simulink library "tqr"  (R2021b)
settings: Solver=VariableStepAuto  StartTime=0.0  StopTime=10.0  RelTol=1e-3
undefined symbols (not defined in the file or in its folder): ATQR_AltRDCActiveFEDUInc_X_pct, ATQR_AltRDCActiveFEDUInc_Y_enum, ATQR_AltRDCActiveFEDUTs_X_pct, ATQR_AltRDCActiveFEDUTs_Y_enum, ATQR_AltRDCActiveREDUInc_X_pct, ATQR_AltRDCActiveREDUInc_Y_enum, ATQR_AltRDCActiveREDUTs_X_pct, ATQR_AltRDCActiveREDUTs_Y_enum, ATQR_CreepFEDUTqIncSR_X_rpm, ATQR_CreepFEDUTqIncSR_Y_Nm, ATQR_CreepFEDUTs_X_rpm, ATQR_CreepFEDUTs_Y_Nm, ATQR_EcoTqFrIncGain_X_Nm, ATQR_EcoTqFrIncGain_Y_pct, ATQR_EcoTqRrIncGain_X_Nm, ATQR_EcoTqRrIncGain_Y_pct, ATQR_EL1FEDUTqDecSR_Y_Nm, ATQR_EL1FEDUTqIncSR_X_rpm, ATQR_EL1FEDUTqIncSR_Y_pct, ATQR_EL1FEDUTs_X_rpm, ATQR_EL1FEDUTs_Y_Nm, ATQR_EL1REDUTqDecSR_Y_Nm, ATQR_EL1REDUTs_Y_Nm, ATQR_FEDUEL1RegenTs_X_rpm, ATQR_FEDUTIPOutTs_X_rpm, ATQR_FrNegRateLimitIncN_X_rpm, ATQR_FrNegRateLimitIncN_Y_Nm, ATQR_FrPosRateLimitIncN_X_rpm, ATQR_FrPosRateLimitIncN_Y_Nm, ATQR_FShaftSpdTqLimCoe_X_rpm, ATQR_FTimerTqLimCoe_X_s, ATQR_FTqZeroTransUpBoundN_X_rpm, ATQR_NL1FEDUTqDecSR_Y_Nm, ATQR_NL1FEDUTqIncSR_X_rpm, ATQR_NL1FEDUTqIncSR_Y_pct, ATQR_NL1FEDUTs_X_rpm, ATQR_NL1FEDUTs_Y_Nm, ATQR_NL1REDUTqDecSR_Y_Nm, ATQR_NL1REDUTs_Y_Nm, ATQR_NormalTqFrIncGain_X_Nm, ATQR_NormalTqFrIncGain_Y_pct, ATQR_NormalTqRrIncGain_X_Nm, ATQR_NormalTqRrIncGain_Y_pct, ATQR_RrNegRateLimitIncN_X_rpm, ATQR_RrNegRateLimitIncN_Y_Nm, ATQR_RrPosRateLimitIncN_X_rpm, ATQR_RrPosRateLimitIncN_Y_Nm, ATQR_RShaftSpdTqLimCoe_X_rpm, ATQR_RTimerTqLimCoe_X_s, ATQR_SL1FEDUTqDecSR_Y_Nm, ATQR_SL1FEDUTqIncSR_X_rpm, ATQR_SL1FEDUTqIncSR_Y_pct, ATQR_SL1FEDUTs_X_rpm, ATQR_SL1FEDUTs_Y_Nm, ATQR_SL1REDUTqDecSR_Y_Nm, ATQR_SL1REDUTs_Y_Nm, ATQR_SportTqFrIncGain_X_Nm, ATQR_SportTqFrIncGain_Y_pct, ATQR_SportTqRrIncGain_X_Nm, ATQR_SportTqRrIncGain_Y_pct ... (+287)
libraries: hcu_lib x19, simulink x17, $bdroot x3
(part 3 of 10)

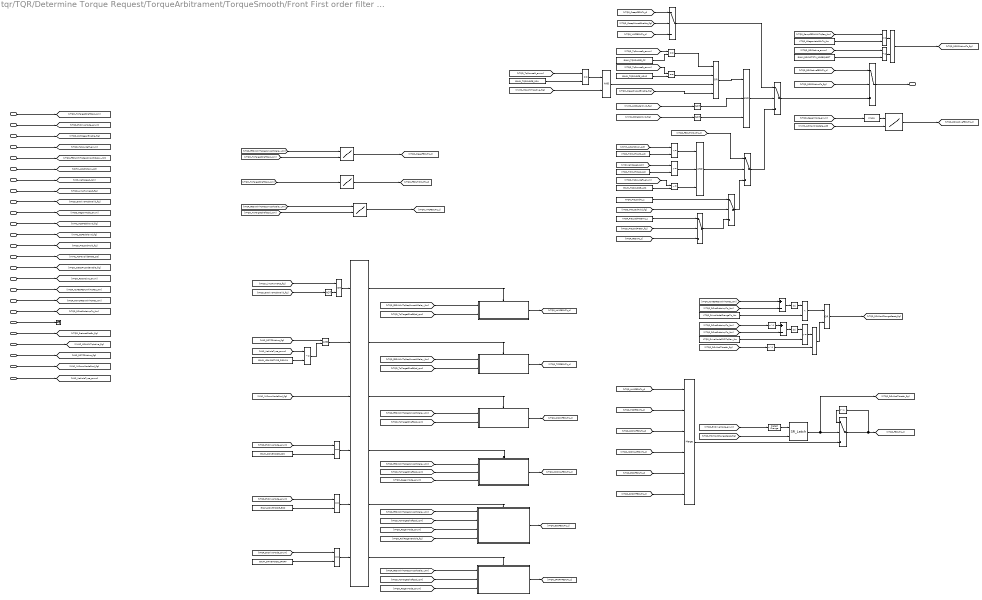
== system tqr/TQR/Determine Torque Request/TorqueArbitrament/TorqueSmooth/Front First order filter input tau map and determination ==
  VTQD_TqTargetShaftSpd_rpm : Inport
  VTQR_EVDriveMode_enum : Inport  Port=2
  VTQD_RollRegenEnable_flg : Inport  Port=3
  VTQD_TqSourceFr_enum : Inport  Port=4
  VTQR_FEDUWhlTqReqSmoothDelay_Nm : Inport  Port=5
  VDHP_ActAPSPosn_pct : Inport  Port=6
  VINP_VehSpeed_kph : Inport  Port=7
  VTQD_LimpHomeAct_flg : Inport  Port=8
  VTQD_EVDriveModeValid_flg : Inport  Port=9
  VTQD_RegenMode_enum : Inport  Port=10
  VVMC_ACCPedalOvrd_flg : Inport  Port=11
  VVMC_CCPedalOvrd_flg : Inport  Port=12
  VTQD_PreLoadHold_flg : Inport  Port=13
  VVMC_ActMaxSlideRate_pct : Inport  Port=14
  VTQD_CreepPrLoadEnable_flg : Inport  Port=15
  VTQD_RDCActive_enum : Inport  Port=16
  VTQR_NoABSFEDUWhlTqReq_Nm : Inport  Port=17
  VTQR_RampFEDUWhlTqReq_Nm : Inport  Port=18
  VTQR_FrFirstOrderInpTq_Nm : Inport  Port=19
  VTQD_PedAccTqEn_flg : Inport  Port=20
  VTQD_PreLoadPreEn_flg : Inport  Port=21
  VVMC_MSAWhlTqActive_flg : Inport  Port=22
  VINP_FrPTCSActive_flg : Inport  Port=23
  VINP_IVISnowModeCmd_flg : Inport  Port=24
  VINP_VehicleType_enum : Inport  Port=25
  AND : Logic  AllPortsSameDT=off  OutDataTypeStr=boolean
  AND1 : Logic  Inputs=3  AllPortsSameDT=off  OutDataTypeStr=boolean
  AND2 : Logic  Inputs=3  AllPortsSameDT=off  OutDataTypeStr=boolean
  AND3 : Logic  AllPortsSameDT=off  OutDataTypeStr=boolean
  AND4 : Logic  AllPortsSameDT=off  OutDataTypeStr=boolean
  Abs : Abs
  Abs4 : Abs
  Add : Sum  Inputs=+-
  Add1 : Sum  Inputs=+-
  Constant : Constant  Value=ENUM_VEHICLETYPE_D31L24
  Constant1 : Constant  Value=ENUM_TQSOURCE_APS
  Constant11 : Constant  Value=ENUM_DRIVEMODE_ECO
  Constant12 : Constant  Value=ENUM_DRIVEMODE_NRM
  Constant16 : Constant  Value=ENUM_DRIVEMODE_SPORT
  Constant2 : Constant  Value=KTQR_DriveModeCMDTqDev_Nm
  Constant3 : Constant  Value=ENUM_TQSOURCE_CC
  Constant32 : Constant  Value=KTQR_TIPOutTsAPS_pct
  Constant33 : Constant  Value=KTQR_TIPOutTsSpd_kph
  Constant34 : Constant  Value=ENUM_TQSOURCE_ADAS
  Constant4 : Constant  Value=KTQR_PreLoadTs_c
  Constant5 : Constant  Value=KTQR_ARegenLatchEnTq_Nm
  Constant6 : Constant  Value=KTQR_PreLoadPreEnTs_c
  Constant7 : Constant  Value=ENUM_RDCACTSTA_NOREQUEST
  Constant8 : Constant  Value=KTQR_DriveModeChangeTq_Nm
  Constant9 : Constant  Value=ENUM_TQSOURCE_MSA
  Data Type Conversion : DataTypeConversion  OutDataTypeStr=single
  Delay : Delay  DelayLength=1
  Delay1 : Delay  DelayLength=1
  Delay2 : Delay  DelayLength=1
  Detect Change : simulink/Logic and Bit Operations/Detect Change  vinit=0  OutDataTypeStr=boolean
  Equal : RelationalOperator  Operator=~=  OutDataTypeStr=boolean  RndMeth=Simplest
  Equal10 : RelationalOperator  Operator===  OutDataTypeStr=boolean  RndMeth=Simplest
  Equal11 : RelationalOperator  Operator===  OutDataTypeStr=boolean  RndMeth=Simplest
  Equal2 : RelationalOperator  Operator=~=  OutDataTypeStr=boolean  RndMeth=Simplest
  Equal9 : RelationalOperator  Operator===  OutDataTypeStr=boolean  RndMeth=Simplest
  GreaterThan2 : RelationalOperator  OutDataTypeStr=boolean  RndMeth=Simplest
  If : If  NumInputs=6  IfExpression=u1~= 0  ElseIfExpressions=u2 ~= 0, u3 ~= 0,u4 ~= 0,u5 ~= 0
  Less Than2 : RelationalOperator  Operator=<=  OutDataTypeStr=boolean  RndMeth=Simplest
  Logical Operator : Logic  AllPortsSameDT=off  OutDataTypeStr=boolean
  Logical Operator14 : Logic  Operator=OR  Inputs=4  AllPortsSameDT=off  OutDataTypeStr=boolean
  Logical Operator2 : Logic  Operator=OR  AllPortsSameDT=off  OutDataTypeStr=boolean
  Logical Operator3 : Logic  Operator=NOT  AllPortsSameDT=off  OutDataTypeStr=boolean
  MTQR_AltRDCActiveFEDUTs_Z_c : Lookup_n-D  BreakpointsForDimension1=ATQR_AltRDCActiveFEDUTs_Y_enum  BreakpointsForDimension2=ATQR_AltRDCActiveFEDUTs_X_pct  Table=MTQR_AltRDCActiveFEDUTs_Z_c  TableDataTypeStr=Inherit: Inherit from 'Table data'  ExtrapMethod=Clip  InternalRulePriority=Speed  RndMeth=Simplest  InputSameDT=on
      settings: InputPortMap=u0,u1
  MTQR_CreepFEDUTs_Z_c : Lookup_n-D  BreakpointsForDimension1=ATQR_CreepFEDUTs_Y_Nm  BreakpointsForDimension2=ATQR_CreepFEDUTs_X_rpm  Table=MTQR_CreepFEDUTs_Z_c  ExtrapMethod=Clip  InternalRulePriority=Speed  RndMeth=Simplest  InputSameDT=on
      settings: InputPortMap=u0,u1
  MTQR_FEDUTIPOutTs_Y_c : Lookup_n-D  NumberOfTableDimensions=1  BreakpointsForDimension1=ATQR_FEDUTIPOutTs_X_rpm  Table=MTQR_FEDUTIPOutTs_Y_c  ExtrapMethod=Clip  InternalRulePriority=Speed  RndMeth=Simplest  InputSameDT=on
  MTQR_VMCFEDUTs_Z_c : Lookup_n-D  BreakpointsForDimension1=ATQR_VMCFEDUTs_Y_Nm  BreakpointsForDimension2=ATQR_VMCFEDUTs_X_rpm  Table=MTQR_VMCFEDUTs_Z_c  ExtrapMethod=Clip  InternalRulePriority=Speed  RndMeth=Simplest  InputSameDT=on
      settings: InputPortMap=u0,u1
  Merge : Merge  Inputs=6
  NOT : Logic  Operator=NOT  AllPortsSameDT=off  OutDataTypeStr=boolean
  NOT1 : Logic  Operator=NOT  AllPortsSameDT=off  OutDataTypeStr=boolean
  OR2 : Logic  Operator=OR  AllPortsSameDT=off  OutDataTypeStr=boolean
  Relational Operator1 : RelationalOperator  Operator=~=  OutDataTypeStr=boolean  RndMeth=Simplest
  Relational Operator2 : RelationalOperator  Operator=<=  OutDataTypeStr=boolean  RndMeth=Simplest
  Relational Operator3 : RelationalOperator  Operator===  OutDataTypeStr=boolean  RndMeth=Simplest
  Relational Operator4 : RelationalOperator  Operator===  OutDataTypeStr=boolean  RndMeth=Simplest
  Relational Operator5 : RelationalOperator  Operator=<  OutDataTypeStr=boolean  RndMeth=Simplest
  Relational Operator6 : RelationalOperator  OutDataTypeStr=boolean  RndMeth=Simplest
  Relational Operator7 : RelationalOperator  Operator===  OutDataTypeStr=boolean  RndMeth=Simplest
  SR_Latch1 : hcu_lib/Basic_Blocks/SR_Latch
  Switch : Switch  Criteria=u2 ~= 0
  Switch1 : Switch  Criteria=u2 ~= 0  Threshold=0.5
  Switch13 : Switch  Criteria=u2 ~= 0
  Switch2 : Switch  Criteria=u2 ~= 0
  Switch3 : Switch  Criteria=u2 ~= 0  Threshold=0.5
  Switch4 : Switch  Criteria=u2 > Threshold
  Switch5 : Switch  Criteria=u2 > Threshold
  Terminator : Terminator
  VTQR_ECOFEDUTs_c : Subsystem  TreatAsAtomicUnit=on
  VTQR_LHMFEDUTs_c : Subsystem  AncestorBlock=tqr_20221220/TQR/Determine Torque Request/TorqueArbitrament/TorqueSmooth/VTQR_LHMFEDUTs_c  TreatAsAtomicUnit=on
  VTQR_NORMALFEDUTs_c : Subsystem  TreatAsAtomicUnit=on
  VTQR_SNOWFEDUTs_c : Subsystem  TreatAsAtomicUnit=on
  VTQR_SPORTFEDUTs_c : Subsystem  AncestorBlock=tqr_20221220/TQR/Determine Torque Request/TorqueArbitrament/TorqueSmooth/VTQR_SPORTFEDUTs_c  TreatAsAtomicUnit=on
  VTQR_TCSFEDUTs_c : Subsystem  TreatAsAtomicUnit=on
  VTQR_FrFirstOrderInpTs_c : Outport
  wires:
  [VTQD_TqTargetShaftSpd_rpm] -> MTQR_FEDUTIPOutTs_Y_c/1
  MTQR_FEDUTIPOutTs_Y_c/1 -> [VTQR_FEDUTIPOutTs_c]  "VTQR_FEDUTIPOutTs_c"
  MTQR_VMCFEDUTs_Z_c/1 -> [VTQR_VMCFEDUTs_c]  "VTQR_VMCFEDUTs_c"
  Constant11/1 -> Equal10/2
  [VTQD_EVDriveModeValid_flg] -> Logical Operator3/1
  Constant12/1 -> Equal11/2
  [VTQR_EVDriveMode_enum] -> Equal11/1
  Constant16/1 -> Equal9/2
  [VTQR_EVDriveMode_enum] -> Equal10/1
  [VTQD_LimpHomeAct_flg] -> Logical Operator2/1
  [VTQR_EVDriveMode_enum] -> Equal9/1
  [VTQR_FEDUWhlTqReqSmoothDelay_Nm] -> VTQR_SPORTFEDUTs_c/1(VTQR_FEDUWhlTqReqSmoothDelay_Nm)
  [VTQD_TqTargetShaftSpd_rpm] -> VTQR_SPORTFEDUTs_c/2(VTQD_TqTargetShaftSpd_rpm)  "VTQD_TqTargetShaftSpd_rpm"
  Logical Operator3/1 -> Logical Operator2/2
  [VTQR_FEDUWhlTqReqSmoothDelay_Nm] -> VTQR_NORMALFEDUTs_c/1(VTQR_FEDUWhlTqReqSmoothDelay_Nm)
  [VTQD_TqTargetShaftSpd_rpm] -> VTQR_NORMALFEDUTs_c/2(VTQD_TqTargetShaftSpd_rpm)  "VTQD_TqTargetShaftSpd_rpm"
  VTQR_LHMFEDUTs_c/1(VTQR_LHMFEDUTs_c) -> [VTQR_LHMFEDUTs_c]
  [VTQR_FEDUWhlTqReqSmoothDelay_Nm] -> VTQR_LHMFEDUTs_c/1(VTQR_FEDUWhlTqReqSmoothDelay_Nm)
  [VTQD_TqTargetShaftSpd_rpm] -> VTQR_LHMFEDUTs_c/2(VTQD_TqTargetShaftSpd_rpm)  "VTQD_TqTargetShaftSpd_rpm"
  [VTQR_FEDUWhlTqReqSmoothDelay_Nm] -> VTQR_ECOFEDUTs_c/1(VTQR_FEDUWhlTqReqSmoothDelay_Nm)
  [VTQD_TqTargetShaftSpd_rpm] -> VTQR_ECOFEDUTs_c/2(VTQD_TqTargetShaftSpd_rpm)  "VTQD_TqTargetShaftSpd_rpm"
  VTQD_TqTargetShaftSpd_rpm/1 -> [VTQD_TqTargetShaftSpd_rpm]
  VTQR_EVDriveMode_enum/1 -> [VTQR_EVDriveMode_enum]
  VTQD_RollRegenEnable_flg/1 -> [VTQD_RollRegenEnable_flg]
  VTQD_TqSourceFr_enum/1 -> [VTQD_TqSourceFr_enum]
  VTQR_FEDUWhlTqReqSmoothDelay_Nm/1 -> [VTQR_FEDUWhlTqReqSmoothDelay_Nm]
  VDHP_ActAPSPosn_pct/1 -> [VDHP_ActAPSPosn_pct]
  VINP_VehSpeed_kph/1 -> [VINP_VehSpeed_kph]
  VTQD_LimpHomeAct_flg/1 -> [VTQD_LimpHomeAct_flg]
  VTQD_EVDriveModeValid_flg/1 -> [VTQD_EVDriveModeValid_flg]
  [VTQD_RegenMode_enum] -> VTQR_NORMALFEDUTs_c/3(VTQD_RegenMode_enum)
  [VTQD_RegenMode_enum] -> VTQR_ECOFEDUTs_c/3(VTQD_RegenMode_enum)
  [VTQD_RegenMode_enum] -> VTQR_SPORTFEDUTs_c/3(VTQD_RegenMode_enum)
  [VTQD_RollRegenEnable_flg] -> VTQR_ECOFEDUTs_c/4(VTQD_RollRegenEnable_flg)
  VTQD_RegenMode_enum/1 -> [VTQD_RegenMode_enum]
  [VTQD_TqTargetShaftSpd_rpm] -> MTQR_VMCFEDUTs_Z_c/2
  [VTQR_FEDUWhlTqReqSmoothDelay_Nm] -> MTQR_VMCFEDUTs_Z_c/1
  [VVMC_CCPedalOvrd_flg] -> NOT1/1
  Switch2/1 -> VTQR_FrFirstOrderInpTs_c/1  "VTQR_FrFirstOrderInpTs_c"
  NOT/1 -> AND1/2
  NOT1/1 -> AND1/3
  [VTQD_CreepPrLoadEnable_flg] -> Logical Operator14/4
  [VVMC_ACCPedalOvrd_flg] -> NOT/1
  AND1/1 -> Switch3/2
  [VTQD_TqSourceFr_enum] -> Relational Operator1/1
  [VTQR_FEDUTIPOutTs_c] -> Switch13/1
  Constant1/1 -> Relational Operator1/2
  AND2/1 -> Switch13/2
  [VINP_VehSpeed_kph] -> GreaterThan2/1
  Constant34/1 -> Relational Operator4/2
  Constant32/1 -> Less Than2/2
  Relational Operator4/1 -> Logical Operator14/2
  [VDHP_ActAPSPosn_pct] -> Less Than2/1
  [VTQD_TqSourceFr_enum] -> Relational Operator3/1
  Less Than2/1 -> AND2/1
  Constant3/1 -> Relational Operator3/2
  Switch13/1 -> Switch3/3
  Constant33/1 -> GreaterThan2/2
  Logical Operator14/1 -> AND1/1
  Relational Operator3/1 -> Logical Operator14/1
  Relational Operator1/1 -> AND2/3
  [VTQD_TqSourceFr_enum] -> Relational Operator4/1
  GreaterThan2/1 -> AND2/2
  VVMC_ACCPedalOvrd_flg/1 -> [VVMC_ACCPedalOvrd_flg]
  VVMC_CCPedalOvrd_flg/1 -> [VVMC_CCPedalOvrd_flg]
  VTQD_PreLoadHold_flg/1 -> [VTQD_PreLoadHold_flg]
  Switch/1 -> Switch13/3
  Constant4/1 -> Switch/1
  [VTQR_VMCFEDUTs_c] -> Switch1/3
  [VTQD_CreepPrLoadEnable_flg] -> Switch1/2
  Switch1/1 -> Switch3/1
  [VTQR_CreepFEDUTs_c] -> Switch1/1
  VTQD_CreepPrLoadEnable_flg/1 -> [VTQD_CreepPrLoadEnable_flg]
  MTQR_CreepFEDUTs_Z_c/1 -> [VTQR_CreepFEDUTs_c]  "VTQR_CreepFEDUTs_c"
  [VTQR_FEDUWhlTqReqSmoothDelay_Nm] -> MTQR_CreepFEDUTs_Z_c/1
  [VTQD_TqTargetShaftSpd_rpm] -> MTQR_CreepFEDUTs_Z_c/2
  VTQD_RDCActive_enum/1 -> [VTQD_RDCActive_enum]
  VTQR_NoABSFEDUWhlTqReq_Nm/1 -> [VTQR_NoABSFEDUWhlTqReq_Nm]
  VTQR_RampFEDUWhlTqReq_Nm/1 -> [VTQR_RampFEDUWhlTqReq_Nm]
  Constant5/1 -> Relational Operator2/2
  Relational Operator2/1 -> AND/1
  AND/1 -> [VTQR_FrRDCActiveTs_flg]  "VTQR_FrRDCActiveTs_flg"
  [VTQR_RDCActiveFEDUTs_c] -> Switch2/1
  [VTQD_RDCActive_enum] -> Equal2/1
  Equal2/1 -> AND/2
  [VTQR_FrRDCActiveTs_flg] -> Switch2/2
  Constant7/1 -> Equal2/2
  [VTQR_RampFEDUWhlTqReq_Nm] -> Relational Operator2/1
  Switch3/1 -> Switch2/3
  VTQR_FrFirstOrderInpTq_Nm/1 -> [VTQR_FrFirstOrderInpTq_Nm]
  [VTQR_FrFirstOrderInpTq_Nm] -> Add/2
  OR2/1 -> [VTQR_FrDrModChangeReset_flg]
  [VTQR_FrDrModTsLatch_flg] -> Delay2/1
  AND4/1 -> OR2/2
  Relational Operator6/1 -> AND4/1
  Delay/1 -> Switch4/1
  Delay2/1 -> AND4/2
  [VTQR_FrDrModChangeReset_flg] -> SR_Latch1/2
  SR_Latch1/1 -> Switch4/2, [VTQR_FrDrModTsLatch_flg]  "VTQR_FrDrModLatch_flg"
  [VTQR_FrFirstOrderInpTq_Nm] -> Add1/2
  Constant8/1 -> Relational Operator5/2
  Switch4/1 -> [VTQR_FEDUTs_c], Delay/1  "VTQR_FEDUTs_c"
  [VTQR_FrFirstOrderInpTq_Nm] -> Delay1/1
  [VTQR_NoABSFEDUWhlTqReq_Nm] -> Add/1
  Delay1/1 -> Add1/1
  Add/1 -> Abs/1
  Abs4/1 -> Relational Operator6/1
  Detect Change/1 -> SR_Latch1/1
  Constant2/1 -> Relational Operator6/2
  Abs/1 -> Relational Operator5/1
  Relational Operator5/1 -> OR2/1
  [VTQR_EVDriveMode_enum] -> Detect Change/1
  Add1/1 -> Abs4/1
  [VTQD_PreLoadHold_flg] -> Switch/2
  Data Type Conversion/1 -> MTQR_AltRDCActiveFEDUTs_Z_c/1
  [VVMC_ActMaxSlideRate_pct] -> MTQR_AltRDCActiveFEDUTs_Z_c/2
  MTQR_AltRDCActiveFEDUTs_Z_c/1 -> [VTQR_RDCActiveFEDUTs_c]  "VTQR_RDCActiveFEDUTs_c"
  [VTQD_RegenMode_enum] -> Data Type Conversion/1
  VVMC_ActMaxSlideRate_pct/1 -> [VVMC_ActMaxSlideRate_pct]
  VTQD_PedAccTqEn_flg/1 -> Terminator/1
  Switch5/1 -> Switch/3
  [VTQR_FEDUTs_c] -> Switch5/3
  [VTQD_PreLoadPreEn_flg] -> Switch5/2
  Constant6/1 -> Switch5/1
  VTQD_PreLoadPreEn_flg/1 -> [VTQD_PreLoadPreEn_flg]
  Relational Operator7/1 -> AND3/1
  [VTQD_TqSourceFr_enum] -> Relational Operator7/1
  VVMC_MSAWhlTqActive_flg/1 -> [VVMC_MSAWhlTqActive_flg]
  [VVMC_MSAWhlTqActive_flg] -> AND3/2
  Constant9/1 -> Relational Operator7/2
  AND3/1 -> Logical Operator14/3
  Logical Operator2/1 -> If/1
  Equal9/1 -> If/6
  Equal10/1 -> If/5
  Equal11/1 -> If/4
  [VINP_IVISnowModeCmd_flg] -> If/3
  If/6 -> VTQR_SPORTFEDUTs_c/Action
  If/5 -> VTQR_ECOFEDUTs_c/Action
  If/4 -> VTQR_NORMALFEDUTs_c/Action
  VTQR_SPORTFEDUTs_c/1(VTQR_SPORTFEDUTs_c) -> [VTQR_SPORTFEDUTs_c]
  VTQR_NORMALFEDUTs_c/1(VTQR_NORMALFEDUTs_c) -> [VTQR_NORMALFEDUTs_c]
  VTQR_ECOFEDUTs_c/1(VTQR_ECOFEDUTs_c) -> [VTQR_ECOFEDUTs_c]
  If/1 -> VTQR_LHMFEDUTs_c/Action
  [VTQD_TqTargetShaftSpd_rpm] -> VTQR_TCSFEDUTs_c/2(VTQD_TqTargetShaftSpd_rpm)
  [VTQR_FEDUWhlTqReqSmoothDelay_Nm] -> VTQR_TCSFEDUTs_c/1(VTQR_FEDUWhlTqReqSmoothDelay_Nm)
  If/2 -> VTQR_TCSFEDUTs_c/Action
  VTQR_TCSFEDUTs_c/1(VTQR_TCSFEDUTs_c) -> [VTQR_TCSFEDUTs_c]  "VTQR_TCSFEDUTs_c"
  [VTQR_FEDUWhlTqReqSmoothDelay_Nm] -> VTQR_SNOWFEDUTs_c/1(VTQR_FEDUWhlTqReqSmoothDelay_Nm)
  [VTQD_TqTargetShaftSpd_rpm] -> VTQR_SNOWFEDUTs_c/2(VTQD_TqTargetShaftSpd_rpm)
  If/3 -> VTQR_SNOWFEDUTs_c/Action
  VTQR_SNOWFEDUTs_c/1(VTQR_SNOWFEDUTs_c) -> [VTQR_SNOWFEDUTs_c]  "VTQR_SNOWFEDUTs_c"
  VINP_FrPTCSActive_flg/1 -> [VINP_FrPTCSActive_flg]
  VINP_IVISnowModeCmd_flg/1 -> [VINP_IVISnowModeCmd_flg]
  [VTQR_SPORTFEDUTs_c] -> Merge/6
  [VTQR_NORMALFEDUTs_c] -> Merge/4
  [VTQR_SNOWFEDUTs_c] -> Merge/3
  [VTQR_TCSFEDUTs_c] -> Merge/2
  [VTQR_ECOFEDUTs_c] -> Merge/5
  [VTQR_LHMFEDUTs_c] -> Merge/1
  Merge/1 -> Switch4/3
  [VINP_VehicleType_enum] -> Equal/1
  Equal/1 -> Logical Operator/2
  Constant/1 -> Equal/2
  [VINP_FrPTCSActive_flg] -> Logical Operator/1
  Logical Operator/1 -> If/2
  VINP_VehicleType_enum/1 -> [VINP_VehicleType_enum]

== system tqr/TQR/Determine Torque Request/TorqueArbitrament/TorqueSmooth/Front Torque zero point transfer boundary map ==
  VTQD_TqTargetShaftSpd_rpm : Inport
  VTQR_EVDriveMode_enum : Inport  Port=2
  Constant1 : Constant  Value=ENUM_DRIVEMODE_ECO
  Constant11 : Constant  Value=ENUM_DRIVEMODE_ECO
  Constant12 : Constant  Value=ENUM_DRIVEMODE_NRM
  Constant16 : Constant  Value=ENUM_DRIVEMODE_SPORT
  Constant2 : Constant  Value=ENUM_DRIVEMODE_NRM
  Constant3 : Constant  Value=ENUM_DRIVEMODE_SPORT
  EcoLow : Subsystem  AncestorBlock=tqr/TQR/Determine Torque Request/TorqueArbitrament/TorqueSmooth/Subsystem/EcoUP
  EcoUP : Subsystem
  Equal{1..5,11} (6 alike) : RelationalOperator  Operator===  OutDataTypeStr=boolean  RndMeth=Simplest
  If1 : If  NumInputs=3  IfExpression=u1~= 0  ElseIfExpressions=u2 ~= 0, u3 ~=0  ShowElse=off
  If2 : If  NumInputs=3  IfExpression=u1~= 0  ElseIfExpressions=u2 ~= 0, u3 ~=0  ShowElse=off
  Merge : Merge  Inputs=3
  Merge1 : Merge  Inputs=3
  NormalLow : Subsystem
  NormalUP : Subsystem
  SportLow : Subsystem  AncestorBlock=tqr/TQR/Determine Torque Request/TorqueArbitrament/TorqueSmooth/Subsystem/SportUP
  SportUP : Subsystem
  VTQR_FrTqZeroTransUpBound_Nm : Outport
  VTQR_FrTqZeroTransLowBound_Nm : Outport  Port=2
  wires:
  VTQD_TqTargetShaftSpd_rpm/1 -> [VTQD_TqTargetShaftSpd_rpm]
  VTQR_EVDriveMode_enum/1 -> [VTQR_EVDriveMode_enum]
  Equal11/1 -> If1/1
  [VTQR_EVDriveMode_enum] -> Equal11/1
  Constant12/1 -> Equal11/2
  [VTQR_EVDriveMode_enum] -> Equal1/1
  [VTQR_EVDriveMode_enum] -> Equal2/1
  Equal2/1 -> If1/3
  Constant16/1 -> Equal2/2
  Equal1/1 -> If1/2
  Constant11/1 -> Equal1/2
  [VTQD_TqTargetShaftSpd_rpm] -> NormalUP/1(VTQD_TqTargetShaftSpd_rpm)
  If1/1 -> NormalUP/Action
  If1/2 -> EcoUP/Action
  If1/3 -> SportUP/Action
  [VTQD_TqTargetShaftSpd_rpm] -> EcoUP/1(VTQD_TqTargetShaftSpd_rpm)
  [VTQD_TqTargetShaftSpd_rpm] -> SportUP/1(VTQD_TqTargetShaftSpd_rpm)
  NormalUP/1(VTQR_FrTqZeroTransUpBound_Nm) -> Merge/1
  EcoUP/1(VTQR_FrTqZeroTransUpBound_Nm) -> Merge/2
  SportUP/1(VTQR_FrTqZeroTransUpBound_Nm) -> Merge/3
  [VTQD_TqTargetShaftSpd_rpm] -> NormalLow/1(VTQD_TqTargetShaftSpd_rpm)
  EcoLow/1(VTQR_FrTqZeroTransLowBound_Nm) -> Merge1/2
  SportLow/1(VTQR_FrTqZeroTransLowBound_Nm) -> Merge1/3
  [VTQD_TqTargetShaftSpd_rpm] -> SportLow/1(VTQD_TqTargetShaftSpd_rpm)
  Constant3/1 -> Equal5/2
  Equal3/1 -> If2/2
  Merge1/1 -> VTQR_FrTqZeroTransLowBound_Nm/1  "VTQR_FrTqZeroTransLowBound_Nm"
  Equal4/1 -> If2/1
  Constant1/1 -> Equal3/2
  [VTQR_EVDriveMode_enum] -> Equal5/1
  [VTQR_EVDriveMode_enum] -> Equal3/1
  [VTQR_EVDriveMode_enum] -> Equal4/1
  [VTQD_TqTargetShaftSpd_rpm] -> EcoLow/1(VTQD_TqTargetShaftSpd_rpm)
  NormalLow/1(VTQR_FrTqZeroTransLowBound_Nm) -> Merge1/1
  Constant2/1 -> Equal4/2
  Equal5/1 -> If2/3
  Merge/1 -> VTQR_FrTqZeroTransUpBound_Nm/1  "VTQR_FrTqZeroTransUpBound_Nm"
  If2/1 -> NormalLow/Action
  If2/2 -> EcoLow/Action
  If2/3 -> SportLow/Action

== system tqr/TQR/Determine Torque Request/TorqueArbitrament/TorqueSmooth/Front Torque zero point transfer status determination  ==
  VTQR_FEDUWhlTqReqSmoothDelay_Nm : Inport
  VTQR_FrTqZeroTransUpBound_Nm : Inport  Port=2
  VTQR_FrTqZeroTransLowBound_Nm : Inport  Port=3
  VTQD_CreepPrLoadEnable_flg : Inport  Port=4
  VVMC_ADASActive_flg : Inport  Port=5
  VTQD_PreLoadPreEn_flg : Inport  Port=6
  VTQR_LaunchEn_flg : Inport  Port=7
  VVMC_ACCPedalOvrd_flg : Inport  Port=8
  VVMC_EstSlope_Deg : Inport  Port=9
  VTQD_RegenMode_enum : Inport  Port=10
  VTQD_AfterAvailableTqDemFr_Nm : Inport  Port=11
  VINP_VehSpeed_kph : Inport  Port=12
  AND : Logic  Inputs=4  AllPortsSameDT=off  OutDataTypeStr=boolean
  Constant : Constant  Value=ZERO_FLOAT
  Constant1 : Constant  Value=ENUM_TQZEROTRANS_POSITIVE
  Constant2 : Constant  Value=ENUM_TQZEROTRANS_NEGATIVE
  Constant3 : Constant  Value=ENUM_TQZEROTRANS_NOZEROTRANS
  Constant4 : Constant  Value=KTQR_CreepZeroTransSW_flg
  Constant5 : Constant  Value=ENUM_REGENLEVEL_OPD
  Constant6 : Constant  Value=KTQR_OPDNoZeroTransTq_Nm
  Constant7 : Constant  Value=KTQR_OPDNoZeroTransSpd_kph
  Equal : RelationalOperator  Operator===  OutDataTypeStr=boolean  RndMeth=Simplest
  Logical Operator : Logic  Inputs=7  AllPortsSameDT=off  OutDataTypeStr=boolean
  Logical Operator{1..4} (4 alike) : Logic  Operator=NOT  AllPortsSameDT=off  OutDataTypeStr=boolean
  NOT : Logic  Operator=NOT  AllPortsSameDT=off  OutDataTypeStr=boolean
  NOT3 : Logic  Operator=NOT  AllPortsSameDT=off  OutDataTypeStr=boolean
  OR : Logic  Operator=OR  AllPortsSameDT=off  OutDataTypeStr=boolean
  OR1 : Logic  Operator=OR  AllPortsSameDT=off  OutDataTypeStr=boolean
  Relational Operator : RelationalOperator  Operator=<  OutDataTypeStr=boolean  RndMeth=Simplest
  Relational Operator1 : RelationalOperator  Operator=>  OutDataTypeStr=boolean  RndMeth=Simplest
  Relational Operator2 : RelationalOperator  OutDataTypeStr=boolean  RndMeth=Simplest
  Relational Operator3 : RelationalOperator  Operator=<=  OutDataTypeStr=boolean  RndMeth=Simplest
  Relational Operator4 : RelationalOperator  Operator=<=  OutDataTypeStr=boolean  RndMeth=Simplest
  Relay1 : Relay  OnSwitchValue=KTQD_OPDHoldGradeUp_Deg  OffSwitchValue=KTQD_OPDHoldGradeDown_Deg  OutDataTypeStr=boolean
  Switch : Switch  Criteria=u2 ~= 0
  Switch1 : Switch  Criteria=u2 ~= 0
  VTQR_FrTqZeroTrans_enum : Outport
  wires:
  VTQR_FEDUWhlTqReqSmoothDelay_Nm/1 -> [VTQR_FEDUWhlTqReqSmoothDelay_Nm]
  VTQR_FrTqZeroTransUpBound_Nm/1 -> [VTQR_FrTqZeroTransUpBound_Nm]
  VTQR_FrTqZeroTransLowBound_Nm/1 -> [VTQR_FrTqZeroTransLowBound_Nm]
  VTQD_CreepPrLoadEnable_flg/1 -> [VTQD_CreepPrLoadEnable_flg]
  VVMC_ADASActive_flg/1 -> [VVMC_ADASActive_flg]
  VTQD_PreLoadPreEn_flg/1 -> [VTQD_PreLoadPreEn_flg]
  VTQR_LaunchEn_flg/1 -> [VTQR_LaunchEn_flg]
  VVMC_ACCPedalOvrd_flg/1 -> [VVMC_ACCPedalOvrd_flg]
  Logical Operator2/1 -> OR/1
  [VTQR_LaunchEn_flg] -> Logical Operator4/1
  Relational Operator1/1 -> Logical Operator/2
  Relational Operator2/1 -> Switch1/2
  [VTQR_FrTqZeroTransLowBound_Nm] -> Relational Operator1/2
  OR/1 -> Logical Operator/4
  [VVMC_ACCPedalOvrd_flg] -> OR/2
  Logical Operator/1 -> Switch/2
  Logical Operator4/1 -> Logical Operator/6
  [VTQR_FEDUWhlTqReqSmoothDelay_Nm] -> Relational Operator2/1
  [VVMC_ADASActive_flg] -> Logical Operator2/1
  Switch1/1 -> Switch/1
  Logical Operator3/1 -> Logical Operator/5
  [VTQR_FEDUWhlTqReqSmoothDelay_Nm] -> Relational Operator/1
  Constant3/1 -> Switch/3
  [VTQD_PreLoadPreEn_flg] -> Logical Operator3/1
  [VTQD_CreepPrLoadEnable_flg] -> Logical Operator1/1
  Constant2/1 -> Switch1/3
  Constant1/1 -> Switch1/1
  Relational Operator/1 -> Logical Operator/1
  [VTQR_FrTqZeroTransUpBound_Nm] -> Relational Operator/2
  [VTQR_FEDUWhlTqReqSmoothDelay_Nm] -> Relational Operator1/1
  Constant/1 -> Relational Operator2/2
  Switch/1 -> VTQR_FrTqZeroTrans_enum/1  "VTQR_FrTqZeroTrans_enum"
  OR1/1 -> Logical Operator/3
  Logical Operator1/1 -> OR1/1
  Constant4/1 -> OR1/2
  Constant6/1 -> Relational Operator3/2
  NOT3/1 -> AND/1
  Constant7/1 -> Relational Operator4/2
  NOT/1 -> Logical Operator/7
  Relay1/1 -> NOT3/1
  Relational Operator3/1 -> AND/3
  Relational Operator4/1 -> AND/4
  Equal/1 -> AND/2
  Constant5/1 -> Equal/2
  AND/1 -> NOT/1
  [VVMC_EstSlope_Deg] -> Relay1/1
  [VTQD_RegenMode_enum] -> Equal/1
  [VTQD_AfterAvailableTqDemFr_Nm] -> Relational Operator3/1
  [VINP_VehSpeed_kph] -> Relational Operator4/1
  VINP_VehSpeed_kph/1 -> [VINP_VehSpeed_kph]
  VTQD_AfterAvailableTqDemFr_Nm/1 -> [VTQD_AfterAvailableTqDemFr_Nm]
  VTQD_RegenMode_enum/1 -> [VTQD_RegenMode_enum]
  VVMC_EstSlope_Deg/1 -> [VVMC_EstSlope_Deg]

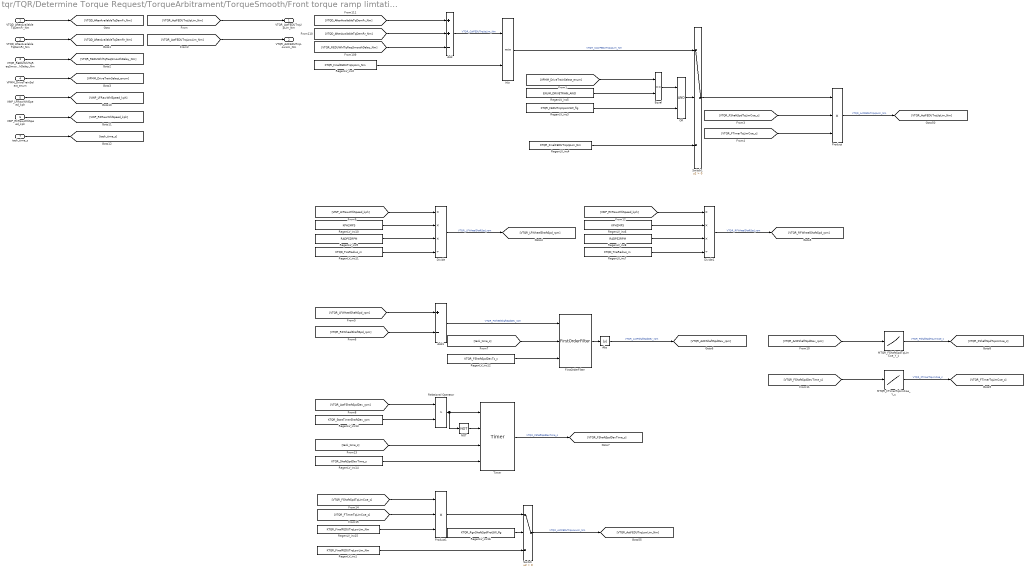
== system tqr/TQR/Determine Torque Request/TorqueArbitrament/TorqueSmooth/Front torque ramp limtation and determination ==
  VTQD_AfterAvailableTqDemFr_Nm : Inport
  VTQD_AfterAvailableTqDemRr_Nm : Inport  Port=2
  VTQR_REDUWhlTqReqSmoothDelay_Nm : Inport  Port=3
  VPMM_DriveTrainSelect_enum : Inport  Port=4
  VINP_LFRawWhlSpeed_kph : Inport  Port=5
  VINP_RFRawWhlSpeed_kph : Inport  Port=6
  task_time_s : Inport  Port=7
  Abs : Abs
  Add : Sum  Inputs=++-
  Add1 : Sum  Inputs=+-
  Divide : Product  Inputs=***/
  Divide1 : Product  Inputs=***/
  Equal : RelationalOperator  Operator===  OutDataTypeStr=boolean  RndMeth=Simplest
  FirstOrderFilter : hcu_lib/Basic_Blocks/FirstOrderFilter
  MTQR_FShaftSpdTqLimCoe_Y_c : Lookup_n-D  NumberOfTableDimensions=1  BreakpointsForDimension1=ATQR_FShaftSpdTqLimCoe_X_rpm  Table=MTQR_FShaftSpdTqLimCoe_Y_c  InternalRulePriority=Speed  RndMeth=Simplest  InputSameDT=on
  MTQR_FTimerTqLimCoe_Y_c : Lookup_n-D  NumberOfTableDimensions=1  BreakpointsForDimension1=ATQR_FTimerTqLimCoe_X_s  Table=MTQR_FTimerTqLimCoe_Y_c  InternalRulePriority=Speed  RndMeth=Simplest  InputSameDT=on
  Min : MinMax  Inputs=2
  NOT : Logic  Operator=NOT  AllPortsSameDT=off  OutDataTypeStr=boolean
  OR : Logic  AllPortsSameDT=off  OutDataTypeStr=boolean
  Product : Product  Inputs=3
  Product1 : Product  Inputs=3
  RegenLV_inc1 : Constant  Value=KTQR_FinalFEDUTrqLowLim_Nm  OutDataTypeStr=single
  RegenLV_inc10 : Constant  Value=KPH2MPS  OutDataTypeStr=single
  RegenLV_inc11 : Constant  Value=KTQD_TireRadius_m  OutDataTypeStr=single
  RegenLV_inc12 : Constant  Value=KTQR_FShaftSpdDevTs_c  OutDataTypeStr=single
  RegenLV_inc13 : Constant  Value=KTQR_StartTimerShaftDev_rpm  OutDataTypeStr=single
  RegenLV_inc14 : Constant  Value=KTQR_ShaftSpdDevTime_s  OutDataTypeStr=single
  RegenLV_inc15 : Constant  Value=KTQR_FinalFEDUTrqLowLim_Nm  OutDataTypeStr=single
  RegenLV_inc16 : Constant  Value=KTQR_RgnShaftSpdProtSW_flg  OutDataTypeStr=single
  RegenLV_inc2 : Constant  Value=KTQR_FinalFEDUTrqUpLim_Nm  OutDataTypeStr=single
  RegenLV_inc3 : Constant  Value=KTQR_FEDUTrqUpLimSW_flg  OutDataTypeStr=single
  RegenLV_inc4 : Constant  Value=KTQR_FinalFEDUTrqUpLim_Nm  OutDataTypeStr=single
  RegenLV_inc5 : Constant  Value=ENUM_DRIVETRAIN_AWD  OutDataTypeStr=single
  RegenLV_inc6 : Constant  Value=KPH2MPS  OutDataTypeStr=single
  RegenLV_inc7 : Constant  Value=KTQD_TireRadius_m  OutDataTypeStr=single
  RegenLV_inc8 : Constant  Value=RADPS2RPM  OutDataTypeStr=single
  RegenLV_inc9 : Constant  Value=RADPS2RPM  OutDataTypeStr=single
  Relational Operator : RelationalOperator  Operator=>  OutDataTypeStr=boolean  RndMeth=Simplest
  Switch : Switch  Criteria=u2 > Threshold
  Switch1 : Switch  Criteria=u2 > Threshold
  Timer : hcu_lib/Basic_Blocks/Timer
  VTQR_ActFEDUTrqUpLim_Nm : Outport
  VTQR_ActFEDUTrqLowLim_Nm : Outport  Port=2
  wires:
  Add/1 -> Min/1  "VTQR_CalFEDUTrqUpLim_Nm"
  RegenLV_inc2/1 -> Min/2
  Min/1 -> Switch1/1  "VTQR_CoorFEDUTrqUpLim_Nm"
  [VTQD_AfterAvailableTqDemFr_Nm] -> Add/1
  [VTQD_AfterAvailableTqDemRr_Nm] -> Add/2
  RegenLV_inc4/1 -> Switch1/3
  VTQD_AfterAvailableTqDemFr_Nm/1 -> [VTQD_AfterAvailableTqDemFr_Nm]
  VTQD_AfterAvailableTqDemRr_Nm/1 -> [VTQD_AfterAvailableTqDemRr_Nm]
  VTQR_REDUWhlTqReqSmoothDelay_Nm/1 -> [VTQR_REDUWhlTqReqSmoothDelay_Nm]
  VPMM_DriveTrainSelect_enum/1 -> [VPMM_DriveTrainSelect_enum]
  [VTQR_REDUWhlTqReqSmoothDelay_Nm] -> Add/3
  [VTQR_ActFEDUTrqLowLim_Nm] -> VTQR_ActFEDUTrqLowLim_Nm/1
  [VTQR_ActFEDUTrqUpLim_Nm] -> VTQR_ActFEDUTrqUpLim_Nm/1
  [VPMM_DriveTrainSelect_enum] -> Equal/1
  RegenLV_inc5/1 -> Equal/2
  RegenLV_inc3/1 -> OR/2
  OR/1 -> Switch1/2
  Equal/1 -> OR/1
  [VTQR_FShaftSpdDevTime_s] -> MTQR_FTimerTqLimCoe_Y_c/1
  MTQR_FTimerTqLimCoe_Y_c/1 -> [VTQR_FTimerTqLimCoe_c]  "VTQR_FTimerTqLimCoe_c"
  Timer/1 -> [VTQR_FShaftSpdDevTime_s]  "VTQR_FShaftSpdDevTime_s"
  [VTQR_RFWheelShaftSpd_rpm] -> Add1/2
  [VTQR_ActFShaftSpdDev_rpm] -> Relational Operator/1
  Relational Operator/1 -> Timer/1, NOT/1
  MTQR_FShaftSpdTqLimCoe_Y_c/1 -> [VTQR_FShaftSpdTqLimCoe_c]  "VTQR_FShaftSpdTqLimCoe_c"
  RegenLV_inc12/1 -> FirstOrderFilter/3
  RegenLV_inc14/1 -> Timer/4
  [task_time_s] -> Timer/3
  RegenLV_inc9/1 -> Divide/3
  RegenLV_inc6/1 -> Divide1/2
  RegenLV_inc10/1 -> Divide/2
  RegenLV_inc13/1 -> Relational Operator/2
  RegenLV_inc8/1 -> Divide1/3
  [VTQR_ActFShaftSpdDev_rpm] -> MTQR_FShaftSpdTqLimCoe_Y_c/1
  Divide/1 -> [VTQR_LFWheelShaftSpd_rpm]  "VTQR_LFWheelShaftSpd_rpm"
  RegenLV_inc7/1 -> Divide1/4
  Divide1/1 -> [VTQR_RFWheelShaftSpd_rpm]  "VTQR_RFWheelShaftSpd_rpm"
  RegenLV_inc11/1 -> Divide/4
  Add1/1 -> FirstOrderFilter/1  "VTQR_FWheelShaftSpdDev_rpm"
  NOT/1 -> Timer/2
  [VTQR_LFWheelShaftSpd_rpm] -> Add1/1
  [task_time_s] -> FirstOrderFilter/2
  Abs/1 -> [VTQR_ActFShaftSpdDev_rpm]  "VTQR_ActFShaftSpdDev_rpm"
  FirstOrderFilter/1 -> Abs/1
  [VINP_LFRawWhlSpeed_kph] -> Divide/1
  [VINP_RFRawWhlSpeed_kph] -> Divide1/1
  VINP_RFRawWhlSpeed_kph/1 -> [VINP_RFRawWhlSpeed_kph]
  task_time_s/1 -> [task_time_s]
  VINP_LFRawWhlSpeed_kph/1 -> [VINP_LFRawWhlSpeed_kph]
  Switch1/1 -> Product/1
  [VTQR_FTimerTqLimCoe_c] -> Product/3
  [VTQR_FShaftSpdTqLimCoe_c] -> Product/2
  Product/1 -> [VTQR_ActFEDUTrqUpLim_Nm]  "VTQR_ActFEDUTrqUpLim_Nm"
  Product1/1 -> Switch/1
  RegenLV_inc16/1 -> Switch/2
  RegenLV_inc1/1 -> Switch/3
  Switch/1 -> [VTQR_ActFEDUTrqLowLim_Nm]  "VTQR_ActFEDUTrqLowLim_Nm"
  RegenLV_inc15/1 -> Product1/3
  [VTQR_FShaftSpdTqLimCoe_c] -> Product1/1
  [VTQR_FTimerTqLimCoe_c] -> Product1/2

== system tqr/TQR/Determine Torque Request/TorqueArbitrament/TorqueSmooth/Front wheel first order filter input torque command determination ==
  VTQR_FrTqZeroTrans_enum : Inport
  VTQR_FrTqZeroTransUpBound_Nm : Inport  Port=2
  VTQR_FrTqZeroTransLowBound_Nm : Inport  Port=3
  VTQD_AfterAvailableTqDemFr_Nm : Inport  Port=4
  VTQR_FrFirstOrderOutTqDelay_Nm : Inport  Port=5
  VTQR_FrGearChange_flg : Inport  Port=6
  VTQR_RampTqCMDGain_c : Inport  Port=7
  AND : Logic  AllPortsSameDT=off  OutDataTypeStr=boolean
  Constant1 : Constant  Value=ZERO_FLOAT
  Constant2 : Constant  Value=KTQR_GearChangeTqSW_flg
  Constant3 : Constant  Value=ENUM_TQZEROTRANS_NOZEROTRANS
  Constant4 : Constant  Value=KTQR_NewRampArchSW_flg
  Constant5 : Constant  Value=ONE_FLOAT
  Product : Product
  Relational Operator : RelationalOperator  Operator===  OutDataTypeStr=boolean  RndMeth=Simplest
  Relational Operator1 : RelationalOperator  OutDataTypeStr=boolean  RndMeth=Simplest
  Relational Operator2 : RelationalOperator  Operator=<=  OutDataTypeStr=boolean  RndMeth=Simplest
  Switch : Switch  Criteria=u2 ~= 0
  Switch1 : Switch  Criteria=u2 ~= 0
  Switch2 : Switch  Criteria=u2 ~= 0
  Switch3 : Switch  Criteria=u2 > Threshold
  Switch4 : Switch  Criteria=u2 > Threshold
  VTQR_FrFirstOrderInpTq_Nm : Outport
  wires:
  [VTQR_FrTqZeroTrans_enum] -> Relational Operator/1
  Constant3/1 -> Relational Operator/2
  Relational Operator/1 -> Switch/2
  Switch1/1 -> Switch/3
  Relational Operator1/1 -> Switch1/2
  [VTQR_FrFirstOrderOutTqDelay_Nm] -> Relational Operator1/1
  [VTQR_FrTqZeroTransUpBound_Nm] -> Relational Operator1/2
  [VTQR_FrTqZeroTransUpBound_Nm] -> Switch1/1
  Switch3/1 -> VTQR_FrFirstOrderInpTq_Nm/1  "VTQR_FrFirstOrderInpTq_Nm"
  [VTQR_FrTqZeroTransLowBound_Nm] -> Switch2/1
  Switch2/1 -> Switch1/3
  [VTQR_FrFirstOrderOutTqDelay_Nm] -> Relational Operator2/1
  [VTQR_FrTqZeroTransLowBound_Nm] -> Relational Operator2/2
  Relational Operator2/1 -> Switch2/2
  [VTQR_FrActRampTqDem_Nm] -> Switch2/3
  VTQR_FrTqZeroTransLowBound_Nm/1 -> [VTQR_FrTqZeroTransLowBound_Nm]
  VTQR_FrTqZeroTrans_enum/1 -> [VTQR_FrTqZeroTrans_enum]
  VTQR_FrFirstOrderOutTqDelay_Nm/1 -> [VTQR_FrFirstOrderOutTqDelay_Nm]
  VTQD_AfterAvailableTqDemFr_Nm/1 -> [VTQD_AfterAvailableTqDemFr_Nm]
  VTQR_FrTqZeroTransUpBound_Nm/1 -> [VTQR_FrTqZeroTransUpBound_Nm]
  VTQR_FrGearChange_flg/1 -> [VTQR_FrGearChange_flg]
  Constant1/1 -> Switch3/1
  Constant2/1 -> AND/2
  [VTQR_FrGearChange_flg] -> AND/1
  AND/1 -> Switch3/2
  Switch/1 -> Switch3/3
  VTQR_RampTqCMDGain_c/1 -> [VTQR_RampTqCMDGain_c]
  Switch4/1 -> Product/2
  [VTQR_RampTqCMDGain_c] -> Switch4/1
  Constant4/1 -> Switch4/2
  Constant5/1 -> Switch4/3
  Product/1 -> [VTQR_FrActRampTqDem_Nm]  "VTQR_FrActRampTqDem_Nm"
  [VTQR_FrActRampTqDem_Nm] -> Switch/1
  [VTQD_AfterAvailableTqDemFr_Nm] -> Product/1
